simulink model "SIMULINK3"  (R2025a)
settings: Solver=ode45  StartTime=0.0  StopTime=10  RelTol=1e-3
model workspace (MAT data in the model file):
  b1 = 1000
  f = 0
  k1 = 16182
  k2 = 19000
  m1 = 290
  m2 = 59
settings Model: Creator=DELL  LastModifiedBy=ernes

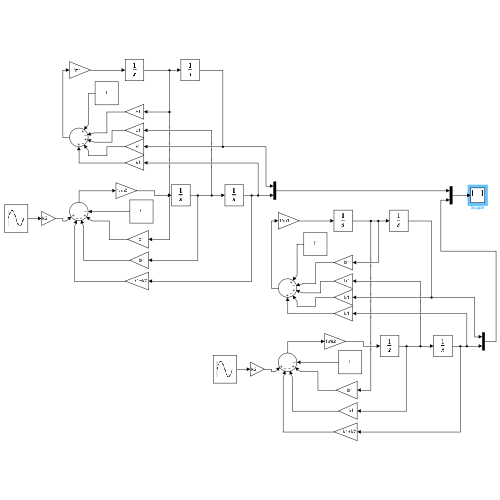
[thumbnail: Simulink's stored preview of the top-level diagram]
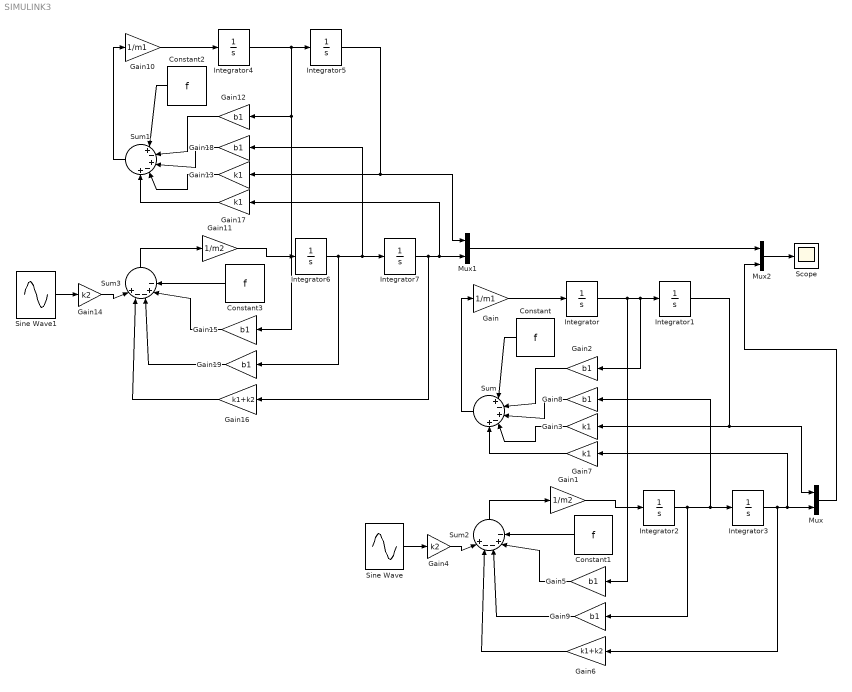
== system SIMULINK3 ==
  Constant{,1..3} (4 alike) : Constant  Value=f
  Gain : Gain  Gain=1/m1
  Gain1 : Gain  Gain=1/m2
  Gain10 : Gain  Gain=1/m1
  Gain11 : Gain  Gain=1/m2
  Gain{2,5,8..9,12,15,18..19} (8 alike) : Gain  Gain=b1
  Gain{3,7,13,17} (4 alike) : Gain  Gain=k1
  Gain14 : Gain  Gain=k2
  Gain16 : Gain  Gain=k1+k2
  Gain4 : Gain  Gain=k2
  Gain6 : Gain  Gain=k1+k2
  Integrator{,1..7} (8 alike) : Integrator
  Mux : Mux  Inputs=2
  Mux1 : Mux  Inputs=2
  Mux2 : Mux  Inputs=2
  Scope : Scope
      settings: ActiveDisplayYMinimum=-0.03544791777641132  ActiveDisplayYMaximum=0.035450816578019712
  Sine Wave : Sin  Amplitude=0.05  Frequency=0.5*pi  SampleTime=0
  Sine Wave1 : Sin  Amplitude=0.05  Frequency=20*pi  SampleTime=0
  Sum : Sum  Inputs=|+-+-+
  Sum1 : Sum  Inputs=|+-+-+
  Sum2 : Sum  Inputs=|+--+-
  Sum3 : Sum  Inputs=|+--+-
  wires:
  Integrator/1 -> Gain2/1, Integrator1/1, Gain5/1
  Gain/1 -> Integrator/1
  Sum/1 -> Gain/1
  Gain1/1 -> Integrator2/1
  Sum2/1 -> Gain1/1
  Integrator1/1 -> Gain3/1, Mux/1
  Mux/1 -> Mux2/2
  Integrator3/1 -> Gain6/1, Gain7/1, Mux/2
  Sine Wave/1 -> Gain4/1
  Constant/1 -> Sum/1
  Integrator2/1 -> Gain9/1, Gain8/1, Integrator3/1
  Gain4/1 -> Sum2/1
  Gain6/1 -> Sum2/2
  Gain3/1 -> Sum/4
  Constant1/1 -> Sum2/5
  Gain7/1 -> Sum/5
  Gain9/1 -> Sum2/3
  Gain2/1 -> Sum/2
  Gain8/1 -> Sum/3
  Gain5/1 -> Sum2/4
  Integrator6/1 -> Gain19/1, Gain18/1, Integrator7/1
  Mux1/1 -> Mux2/1
  Gain14/1 -> Sum3/1
  Gain10/1 -> Integrator4/1
  Constant2/1 -> Sum1/1
  Constant3/1 -> Sum3/5
  Gain18/1 -> Sum1/3
  Gain19/1 -> Sum3/3
  Gain17/1 -> Sum1/5
  Gain13/1 -> Sum1/4
  Gain15/1 -> Sum3/4
  Gain11/1 -> Integrator6/1
  Sum3/1 -> Gain11/1
  Sum1/1 -> Gain10/1
  Integrator5/1 -> Gain13/1, Mux1/1
  Integrator7/1 -> Gain16/1, Gain17/1, Mux1/2
  Integrator4/1 -> Gain12/1, Gain15/1, Integrator5/1
  Gain12/1 -> Sum1/2
  Gain16/1 -> Sum3/2
  Sine Wave1/1 -> Gain14/1
  Mux2/1 -> Scope/1
